simulink library "MainCANRX"  (R2015b)
settings: Solver=ode1  StartTime=0.0  StopTime=Inf  FixedStep=0.001  RelTol=1e-3
PostLoadFcn:
  | , if any(exist('dsrtsu_mdlpostloadfcn', 'file') == [2, 3, 6]), try dsrtsu_mdlpostloadfcn('Execute', bdroot); catch fprintf('Error in PostLoadFcn (dsrtsu_mdlpostloadfcn) for model "%s":\n %s\n', bdroot, lasterr); end, end,
libraries: rtican x4
settings Model: DSRTSU_INTERNAL_RTI_VER=460  DSRTSU_INTERNAL_RTI_TYPE=rti1401  Creator=luis  LastModifiedBy=luis
settings OptimizationCC: BlockReduction=off  OptimizeBlockIOStorage=off  BufferReuse=off  GlobalBufferReuse=off  ExpressionFolding=off  LocalBlockOutputs=off
settings HardwareCC: ProdEndianess=BigEndian  ProdWordSize=32  ProdHWDeviceType=Generic->Custom  TargetIntDivRoundTo=Zero  TargetEndianess=BigEndian  TargetHWDeviceType=Generic->Custom
settings RTWCC: SystemTargetFile=rti1401.tlc  MakeCommand=make_rti  TemplateMakefile=rti1401.tmf  Description=dSPACE DS1401 Hardware Platform
settings STFCustomTargetCC: ParMdlRefBuildCompliant=on  ConcurrentExecutionCompliant=off  GeneratePreprocessorConditionals=Use local settings  MatFileLogging=on  CPPClassGenCompliant=off  SystemTargetFile=rti1401.tlc
settings GRTTargetCC: CompOptLevelCompliant=off  ConcurrentExecutionCompliant=off  CombineOutputUpdateFcns=off  CPPClassGenCompliant=off  GRTInterface=on  UseToolchainInfoCompliant=off

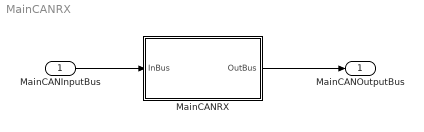
== system MainCANRX ==
  MainCANInputBus : Inport
  MainCANRX : Subsystem
  MainCANOutputBus : Outport
  wires:
  MainCANInputBus/1 -> MainCANRX/1(InBus)
  MainCANRX/1(OutBus) -> MainCANOutputBus/1

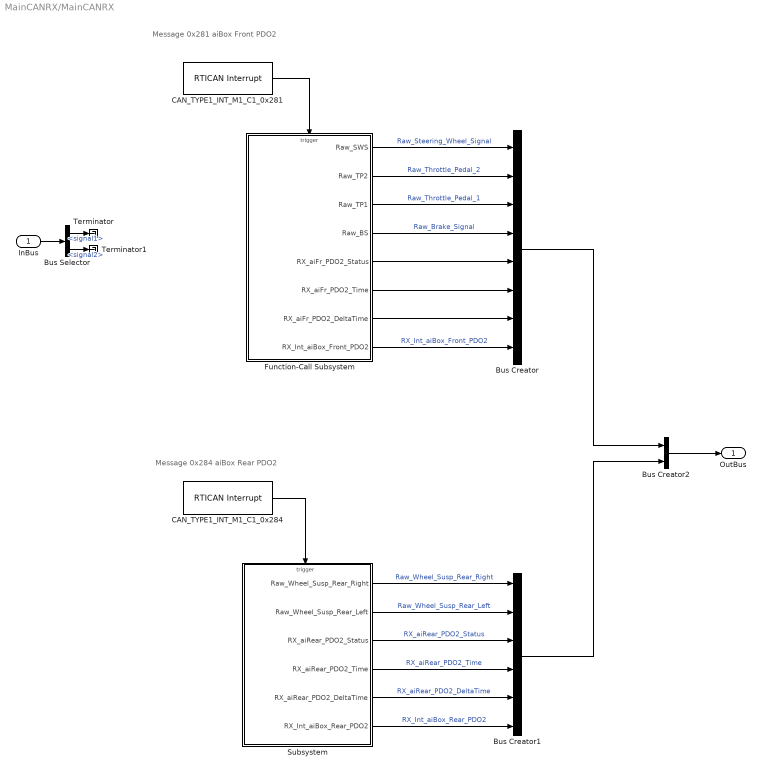
== system MainCANRX/MainCANRX ==
  note: Message 0x284 aiBox Rear PDO2
  note: Message 0x281 aiBox Front PDO2
  InBus : Inport
  Bus Creator : BusCreator  Inputs=8
  Bus Creator1 : BusCreator  Inputs=6
  Bus Creator2 : BusCreator  Inputs=2
  Bus Selector : BusSelector  OutputSignals=signal1,signal2
  CAN_TYPE1_INT_M1_C1_0x281 : rtican/RTICAN Interrupt  Reserved1=[]  Reserved2=[]  Reserved3=[]  Reserved4=[]  BoardTypeNo=[]  BoardNo=[]  ChannelNo=[]  Parameters=[]  InterruptName=[]  BoardIntNo=[]  Sfcn_Int_Struct=[]  BoardType=[]  SintNo=[]  Int_Struct=[]  DialogFcn=[]  UnitName=[]  Revision=[]  UnitValues=[]  DSProperties=struct('RTI',struct('Version',uint32(4),'BlockType',struct('isSLSource',uint8(1),'isSLSink',uint8(0),'isHWSource',uint8(1),'isHWSink',uint8(0),'isSetup',uint8(0),'isInline',uint8(1),'isNonInline',uint8(0),'isInterrupt',uint8(1),'isChannelwise',uint8(0)),'IOBoardType','RTICAN','UnitType','HWINT','Identifier','CANINT','DialogType','ML','BlockSet','RTICAN','RelationId',struct('TH',struct('BlockId','HWINT')),'SlaveProcessor','CAN'))  RTIBlockInterface=struct('OutputPortsWidth',int32(1),'FunctionCall',uint32(0),'OutputPortsActive',1,'DialogFcn','rtican_interrupt_gui','BlockDisplay',{{['CAN RX Interrupt'],'center'}},'IconTransparency','off','ParameterTunableNames',{{}},'InitLevel',3,'BlockName',struct('Token',{{'CAN_TYPE','_INT_M','_C'}},'BlockParam',{{'BoardTypeNo','BoardNo','ChannelNo'}}),'Options',{{'SS_OPTION_FORCE_NONINLINED_FCNCALL','SS_OPTION_ASYNCHRONOUS_INTERRUPT'}})  RTIBlockParameters=struct('BoardTypeNo',{{1,'OFF',[]}},'BoardNo',{{1,'ON',[1 16]}},'ChannelNo',{{1,'ON',[1 2]}},'Parameters',{{struct('general',struct('Type','RX','NumFormat','hex','MsgIdFormat','STD','MsgId',641,'isFromLib',0)),'OFF',[]}},'GroupId',{{struct('Group','RTICAN','No',1,'Behavior','NAMECHANGE','BlockType','SINK','NameChangeFlag',0),'OFF',[]}},'SFcnRTICANInterrupt',{{0,'OFF',[]}},'ThSrcSgnName',{{['CAN_TYPE1_M1_C1 RX Interrupt'],'OFF',[]}},'ThBlk',{{['struct(''blkh'',[''mainECU/MainCAN RX/CAN_TYPE1_INT_M1_C1_0x281''],''srcId'',''CAN1'',''srcSgnId'',''CAN1'',''intervalTmrBlockId'',[],''srcSgnName'',[''CAN_TYPE1_M1_C1 RX Interrupt''],''srcCpuId'','''',''isSrcCpu'',1,''isTargetCpu'',1,''srcOnMasterCpu'',1,''boardType'',''CAN'',''boardTypeNo'',''1'',''boardNo'',0,''intNo'',0,''subIntNo'',-1,''period'',0,''entryPoint'',''rti_CAN1'',''blockName'',''CAN_TYPE1_INT_M1_C1_0x281'',''taskNameDisplayExt'','''',''taskType'',''HWINT'',''groupId'',''CANINT1B1'',''hookFcn'',''NULL'',''isTimerTaskSrc'',0,''service'','''',''mpBlkId'','''',''taskPriorityPreConfig'',''none'',''taskPriority'',-1,''taskSortWeighting'',[],''taskSchedulingPolicy'',''FCFS'',''taskOvrPreConfig'',''none'',''taskOvrStrategy'',1,''taskOvrQueueSize'',1,''taskVisibility'',''on'',''taskGroupId'','''',''taskGroupDisplayOrder'',[],''serviceDynamicGen'',0,''disableCodeGen'',0,''boardBase'',''0'',''noBoardBase'','''')'],'OFF',[]}},'PHSBoardBaseId',{{'DS4302','OFF',[]}},'TLCFileName',{{'rtican_interrupt','OFF',[]}})  RTISFcnParameters=struct('SFcnRTICANInterrupt','struct','ThBlk','struct','PHSBoardBaseId','char','TLCFileName','char')  RTIBlockParaDefault=struct('BoardTypeNo',4302,'BoardNo',1,'ChannelNo',1,'Parameters',struct('general',struct('Type','RX','NumFormat','dec','MsgIdFormat','STD','MsgId',100,'isFromLib',1)),'GroupId',struct('Group',{{'RTICAN'}},'No',1,'Behavior',{{'NAMECHANGE'}},'BlockType',{{'SINK'}},'NameChangeFlag',0),'SFcnRTICANInterrupt',0,'ThSrcSgnName',['DS4302CAN_B1_C1 RX Interrupt'],'ThBlk',['struct(''srcSgnId'', '''')'],'PHSBoardBaseId','DS4302','TLCFileName','rtican_interrupt')
      settings: AttributesFormatString=Group Id: RTICAN1\n
  CAN_TYPE1_INT_M1_C1_0x284 : rtican/RTICAN Interrupt  Reserved1=[]  Reserved2=[]  Reserved3=[]  Reserved4=[]  BoardTypeNo=[]  BoardNo=[]  ChannelNo=[]  Parameters=[]  InterruptName=[]  BoardIntNo=[]  Sfcn_Int_Struct=[]  BoardType=[]  SintNo=[]  Int_Struct=[]  DialogFcn=[]  UnitName=[]  Revision=[]  UnitValues=[]  DSProperties=struct('RTI',struct('Version',uint32(4),'BlockType',struct('isSLSource',uint8(1),'isSLSink',uint8(0),'isHWSource',uint8(1),'isHWSink',uint8(0),'isSetup',uint8(0),'isInline',uint8(1),'isNonInline',uint8(0),'isInterrupt',uint8(1),'isChannelwise',uint8(0)),'IOBoardType','RTICAN','UnitType','HWINT','Identifier','CANINT','DialogType','ML','BlockSet','RTICAN','RelationId',struct('TH',struct('BlockId','HWINT')),'SlaveProcessor','CAN'))  RTIBlockInterface=struct('OutputPortsWidth',int32(1),'FunctionCall',uint32(0),'OutputPortsActive',1,'DialogFcn','rtican_interrupt_gui','BlockDisplay',{{['CAN RX Interrupt'],'center'}},'IconTransparency','off','ParameterTunableNames',{{}},'InitLevel',3,'BlockName',struct('Token',{{'CAN_TYPE','_INT_M','_C'}},'BlockParam',{{'BoardTypeNo','BoardNo','ChannelNo'}}),'Options',{{'SS_OPTION_FORCE_NONINLINED_FCNCALL','SS_OPTION_ASYNCHRONOUS_INTERRUPT'}})  RTIBlockParameters=struct('BoardTypeNo',{{1,'OFF',[]}},'BoardNo',{{1,'ON',[1 16]}},'ChannelNo',{{1,'ON',[1 2]}},'Parameters',{{struct('general',struct('Type','RX','NumFormat','hex','MsgIdFormat','STD','MsgId',644,'isFromLib',0)),'OFF',[]}},'GroupId',{{struct('Group','RTICAN','No',1,'Behavior','NAMECHANGE','BlockType','SINK','NameChangeFlag',0),'OFF',[]}},'SFcnRTICANInterrupt',{{0,'OFF',[]}},'ThSrcSgnName',{{['CAN_TYPE1_M1_C1 RX Interrupt'],'OFF',[]}},'ThBlk',{{['struct(''blkh'',[''mainECU/MainCAN RX/CAN_TYPE1_INT_M1_C1_0x284''],''srcId'',''CAN2'',''srcSgnId'',''CAN2'',''intervalTmrBlockId'',[],''srcSgnName'',[''CAN_TYPE1_M1_C1 RX Interrupt''],''srcCpuId'','''',''isSrcCpu'',1,''isTargetCpu'',1,''srcOnMasterCpu'',1,''boardType'',''CAN'',''boardTypeNo'',''1'',''boardNo'',0,''intNo'',1,''subIntNo'',-1,''period'',0,''entryPoint'',''rti_CAN2'',''blockName'',''CAN_TYPE1_INT_M1_C1_0x284'',''taskNameDisplayExt'','''',''taskType'',''HWINT'',''groupId'',''CANINT1B1'',''hookFcn'',''NULL'',''isTimerTaskSrc'',0,''service'','''',''mpBlkId'','''',''taskPriorityPreConfig'',''none'',''taskPriority'',-1,''taskSortWeighting'',[],''taskSchedulingPolicy'',''FCFS'',''taskOvrPreConfig'',''none'',''taskOvrStrategy'',1,''taskOvrQueueSize'',1,''taskVisibility'',''on'',''taskGroupId'','''',''taskGroupDisplayOrder'',[],''serviceDynamicGen'',0,''disableCodeGen'',0,''boardBase'',''0'',''noBoardBase'','''')'],'OFF',[]}},'PHSBoardBaseId',{{'DS4302','OFF',[]}},'TLCFileName',{{'rtican_interrupt','OFF',[]}})  RTISFcnParameters=struct('SFcnRTICANInterrupt','struct','ThBlk','struct','PHSBoardBaseId','char','TLCFileName','char')  RTIBlockParaDefault=struct('BoardTypeNo',4302,'BoardNo',1,'ChannelNo',1,'Parameters',struct('general',struct('Type','RX','NumFormat','dec','MsgIdFormat','STD','MsgId',100,'isFromLib',1)),'GroupId',struct('Group',{{'RTICAN'}},'No',1,'Behavior',{{'NAMECHANGE'}},'BlockType',{{'SINK'}},'NameChangeFlag',0),'SFcnRTICANInterrupt',0,'ThSrcSgnName',['DS4302CAN_B1_C1 RX Interrupt'],'ThBlk',['struct(''srcSgnId'', '''')'],'PHSBoardBaseId','DS4302','TLCFileName','rtican_interrupt')
      settings: AttributesFormatString=Group Id: RTICAN1\n
  Function-Call Subsystem : Subsystem  TreatAsAtomicUnit=on
  Subsystem : Subsystem
  Terminator : Terminator
  Terminator1 : Terminator
  OutBus : Outport
  wires:
  CAN_TYPE1_INT_M1_C1_0x281/1 -> Function-Call Subsystem/Trigger
  CAN_TYPE1_INT_M1_C1_0x284/1 -> Subsystem/Trigger
  Function-Call Subsystem/1(Raw_SWS) -> Bus Creator/1  "Raw_Steering_Wheel_Signal"
  Subsystem/6(RX_Int_aiBox_Rear_PDO2) -> Bus Creator1/6  "RX_Int_aiBox_Rear_PDO2"
  Subsystem/1(Raw_Wheel_Susp_Rear_Right) -> Bus Creator1/1  "Raw_Wheel_Susp_Rear_Right"
  Function-Call Subsystem/8(RX_Int_aiBox_Front_PDO2) -> Bus Creator/8  "RX_Int_aiBox_Front_PDO2"
  Subsystem/3(RX_aiRear_PDO2_Status) -> Bus Creator1/3  "RX_aiRear_PDO2_Status"
  Function-Call Subsystem/3(Raw_TP1) -> Bus Creator/3  "Raw_Throttle_Pedal_1"
  Function-Call Subsystem/7(RX_aiFr_PDO2_DeltaTime) -> Bus Creator/7
  Function-Call Subsystem/6(RX_aiFr_PDO2_Time) -> Bus Creator/6
  Function-Call Subsystem/4("Raw_BS ") -> Bus Creator/4  "Raw_Brake_Signal"
  Subsystem/4(RX_aiRear_PDO2_Time) -> Bus Creator1/4  "RX_aiRear_PDO2_Time"
  Subsystem/2(Raw_Wheel_Susp_Rear_Left) -> Bus Creator1/2  "Raw_Wheel_Susp_Rear_Left"
  Function-Call Subsystem/5(RX_aiFr_PDO2_Status) -> Bus Creator/5
  Function-Call Subsystem/2(Raw_TP2) -> Bus Creator/2  "Raw_Throttle_Pedal_2"
  Subsystem/5(RX_aiRear_PDO2_DeltaTime) -> Bus Creator1/5  "RX_aiRear_PDO2_DeltaTime"
  Bus Selector/1 -> Terminator/1  "<signal1>"
  InBus/1 -> Bus Selector/1
  Bus Creator/1 -> Bus Creator2/1
  Bus Creator1/1 -> Bus Creator2/2
  Bus Creator2/1 -> OutBus/1
  Bus Selector/2 -> Terminator1/1  "<signal2>"

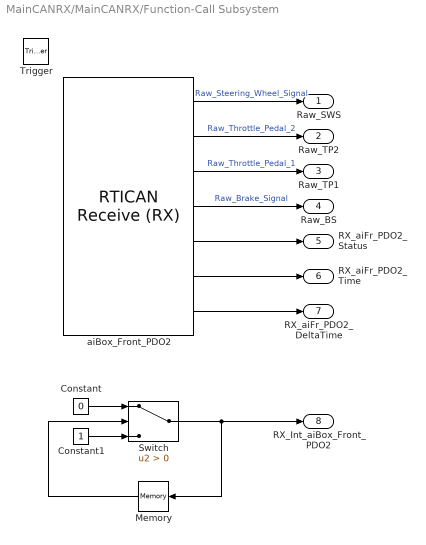
== system MainCANRX/MainCANRX/Function-Call Subsystem ==
  Trigger : TriggerPort  TriggerType=function-call  OutputDataType=double
  Constant : Constant  Value=0
  Constant1 : Constant
  Memory : Memory  InheritSampleTime=on
  Switch : Switch  Criteria=u2 > Threshold
  aiBox_Front_PDO2 : rtican/RTICAN Receive (RX)   Reserved1=[]  Reserved2=[]  Reserved3=[]  Reserved4=[]  SfcnMessage=[]  Msg_Struct=[]  BoardTypeNo=[]  BoardNo=[]  ChannelNo=[]  Parameters=[]  DialogFcn=[]  UnitName=[]  Revision=[]  UnitValues=[]  DSProperties=struct('RTI',struct('Version',uint32(5),'BlockType',struct('isSLSource',uint8(1),'isSLSink',uint8(1),'isHWSource',uint8(0),'isHWSink',uint8(0),'isSetup',uint8(0),'isInline',uint8(1),'isNonInline',uint8(0),'isInterrupt',uint8(0),'isChannelwise',uint8(0)),'IOBoardType','RTICAN','UnitType','MESSAGE','Identifier','RX','DialogType','MSVC','BlockSet','RTICAN','SlaveProcessor','CAN'))  RTIBlockInterface=struct('OutputPortsWidth',int32([1 1 1 1 1 1 1]),'OutputPortsActive',[1 1 1 1 1 1 1],'OutputPortsName',{{'Raw_Steering_Wheel_Signal','Raw_Throttle_Pedal_2','Raw_Throttle_Pedal_1','Raw_Brake_Signal',['RX status'],['RX time'],['RX delta time']}},'OutputPortsDataType',{{'SS_DOUBLE','SS_DOUBLE','SS_DOUBLE','SS_DOUBLE','SS_DOUBLE','SS_DOUBLE','SS_DOUBLE'}},'OutputPortsLabel',{{'Raw_Steering_Wheel_Signal','Raw_Throttle_Pedal_2','Raw_Throttle_Pedal_1','Raw_Brake_Signal','','',''}},'OutputPortsLabelMode','ON','InputPortsWidth',int32(0),'InputPortsActive',0,'DialogFcn','rtican_message_interface_gui','BlockDisplay',{{'','center'}},'IconTransparency','on','ParameterTunableNames',{{}},'InitLevel',3,'BlockName',struct('Token',{{'aiBox_Front_PDO2'}}),'SampleTime',{{-1}},'TriggerPort',{{'none'}},'EnablePort',{{'none'}})  RTIBlockParameters=struct('BoardTypeNo',{{1,'OFF',[]}},'BoardNo',{{1,'ON',[1 16]}},'ChannelNo',{{1,'ON',[1 2]}},'Parameters',{{struct('DataFileSupport',struct('DataFileSelectedMaster',1,'DataFileSelectedLocal',1,'DataFileName',['c:\users\luis\documents\tuc racing\mainecu\database\main_0_2.dbc|'],'DataFileDate',{{{['07-ene.-2017 20:06:27']}}},'SelectedFile','database\main_0_2.dbc'),'Options',struct('StatusSelected',1,'TimeSelected',1,'DeltaTimeSelected',1,'BytePortSelected',0,'MessageLengthSelected',0,'TriggerPort',struct('Selected',0,'TriggerType',0),'UserCoding',struct('Selected',0,'InterfaceFile','UserDecodingFile','FcnName','UserDecodeFcn','InportSelected',0,'InportWidth',1,'OutportSelected',0,'OutportWidth',1),'EnablePortSelected',0,'SignalOnPortnameSelected',1,'UseRXService',0),'Message',struct('MsgOnBlocknameSelected',1,'MsgName','aiBox_Front_PDO2','MsgIdFormat',0,'MsgId',641,'MsgLength',8,'NumSignals',4,'SampleTime',-1,'Signal',struct('SgnName',{'Raw_Steering_Wheel_Signal','Raw_Throttle_Pedal_2','Raw_Throttle_Pedal_1','Raw_Brake_Signal'},'SgnStartBit',{0,16,32,48},'SgnLength',{16,16,16,16},'SgnType',{0,0,0,0},'ModeValue',{-1,-1,-1,-1},'DataType',{0,0,0,0},'ByteLayout',{2,2,2,2},'Factor',{1,1,1,1},'Offset',{0,0,0,0},'SgnComment',{{''},{''},{''},{''}},'SgnUnit',{'','','',''},'Min',{0,0,0,0},'Max',{0,0,0,0},'SLDataType',{'SS_DOUBLE','SS_DOUBLE','SS_DOUBLE','SS_DOUBLE'}),'MsgIdNumFormat',1,'MsgComment',{{''}}),'Version',1.2,'general',struct('isFromLib',0)),'OFF',[]}},'GroupId',{{struct('Group',{{'RTICAN'}},'No',1,'Behavior',{{'NAMECHANGE'}},'BlockType',{{'SINK'}},'NameChangeFlag',0),'OFF',[]}},'SFcnRTICANMessage',{{struct('MsgType','RX','SFcnPortType','Scalar','MsgName','aiBox_Front_PDO2','MsgIdFormat','STD','MsgId',641,'MsgLength',8,'NumSignals',4,'SampleTime',-1,'Signal',struct('SgnName',{'Raw_Steering_Wheel_Signal','Raw_Throttle_Pedal_2','Raw_Throttle_Pedal_1','Raw_Brake_Signal'},'SgnStartBit',{0,16,32,48},'SgnLength',{16,16,16,16},'SgnType',{'standard','standard','standard','standard'},'ModeValue',{-1,-1,-1,-1},'DataType',{['unsigned int'],['unsigned int'],['unsigned int'],['unsigned int']},'ByteLayout',{['motorola back.'],['motorola back.'],['motorola back.'],['motorola back.']},'Factor',{1,1,1,1},'Offset',{0,0,0,0},'SLDataType',{'SS_DOUBLE','SS_DOUBLE','SS_DOUBLE','SS_DOUBLE'}),'StatusSelected','yes','TimeSelected','yes','DeltaTimeSelected','yes','BytePortSelected','no','MessageLengthSelected','no','TriggerPort',struct('Selected','no','TriggerType',0),'UserCoding',struct('Selected','no','InterfaceFile','UserDecodingFile','FcnName','UserDecodeFcn','InportSelected','no','InportWidth',1,'OutportSelected','no','OutportWidth',1),'EnablePortSelected','no','UseRXService','no','BoardType','DS1','BoardNo',1,'ControllerNo',1),'OFF',[]}},'TLCFileName',{{'rtican_rx_message','OFF',[]}})  RTISFcnParameters=struct('SFcnRTICANMessage','struct','TLCFileName','char')  RTIBlockParaDefault=struct('BoardTypeNo',4302,'BoardNo',1,'ChannelNo',1,'Parameters',struct('DataFileSupport',struct('DataFileSelectedMaster',0,'DataFileSelectedLocal',0,'DataFileName','','DataFileDate','','SelectedFile',['<no file selected>']),'Options',struct('StatusSelected',1,'TimeSelected',1,'DeltaTimeSelected',1,'BytePortSelected',0,'MessageLengthSelected',0,'TriggerPort',struct('Selected',0,'TriggerType','rising'),'UserCoding',struct('Selected',0,'InterfaceFile','UserDecodingFile','FcnName','UserDecodeFcn','InportSelected',0,'InportWidth',1,'OutportSelected',0,'OutportWidth',1),'EnablePortSelected',0,'SignalOnPortnameSelected',1,'UseRXService',0),'Message',struct('MsgOnBlocknameSelected',0,'MsgName',['RX Message'],'MsgIdFormat',0,'MsgId',100,'MsgLength',8,'NumSignals',1,'SampleTime',-1,'Signal',struct('SgnName',['RX signal'],'SgnStartBit',0,'SgnLength',8,'SgnType',0,'ModeValue',-1,'DataType',0,'SLDataType','SS_DOUBLE','ByteLayout',0,'Factor',1,'Offset',0,'Min',0,'Max',255,'SgnComment',{{}},'SgnUnit',''),'MsgIdNumFormat',0,'MsgComment',{{''}}),'Version',1.2,'general',struct('isFromLib',1)),'GroupId',struct('Group',{{'RTICAN'}},'No',1,'Behavior',{{'NAMECHANGE'}},'BlockType',{{'SINK'}},'NameChangeFlag',0),'SFcnRTICANMessage',struct('MsgType','RX','MsgName',['RX Message'],'MsgIdFormat','STD','MsgId',100,'MsgLength',8,'NumSignals',1,'SampleTime',-1,'Signal',struct('SgnName',['RX signal'],'SgnStartBit',0,'SgnLength',8,'SgnType','standard','ModeValue',-1,'DataType',['unsigned int'],'ByteLayout',['little endian'],'SLDataType','SS_DOUBLE','Factor',1,'Offset',0),'StatusSelected','yes','TimeSelected','yes','DeltaTimeSelected','yes','BytePortSelected','no','MessageLengthSelected','no','EnablePortSelected','no','UserCoding',struct('Selected','no','InterfaceFile','UserDecodingFile','FcnName','UserDecodeFcn','InportSelected','no','InportWidth',1,'OutportSelected','no','OutportWidth',1),'TriggerPort',struct('Selected','no','TriggerType','rising'),'UseRXService','no','BoardType','DS4302','BoardNo',1,'ControllerNo',1,'SFcnPortType','Scalar'),'TLCFileName','rtican_rx_message')
      settings: AttributesFormatString=Group Id: RTICAN1\n
  Raw_SWS : Outport
  Raw_TP2 : Outport  Port=2
  Raw_TP1 : Outport  Port=3
  "Raw_BS " : Outport  Port=4
  RX_aiFr_PDO2_Status : Outport  Port=5
  RX_aiFr_PDO2_Time : Outport  Port=6
  RX_aiFr_PDO2_DeltaTime : Outport  Port=7
  RX_Int_aiBox_Front_PDO2 : Outport  Port=8
  wires:
  aiBox_Front_PDO2/1 -> Raw_SWS/1  "Raw_Steering_Wheel_Signal"
  aiBox_Front_PDO2/2 -> Raw_TP2/1  "Raw_Throttle_Pedal_2"
  aiBox_Front_PDO2/3 -> Raw_TP1/1  "Raw_Throttle_Pedal_1"
  aiBox_Front_PDO2/4 -> "Raw_BS "/1  "Raw_Brake_Signal"
  aiBox_Front_PDO2/5 -> RX_aiFr_PDO2_Status/1
  aiBox_Front_PDO2/6 -> RX_aiFr_PDO2_Time/1
  aiBox_Front_PDO2/7 -> RX_aiFr_PDO2_DeltaTime/1
  Switch/1 -> Memory/1, RX_Int_aiBox_Front_PDO2/1
  Memory/1 -> Switch/2
  Constant1/1 -> Switch/3
  Constant/1 -> Switch/1

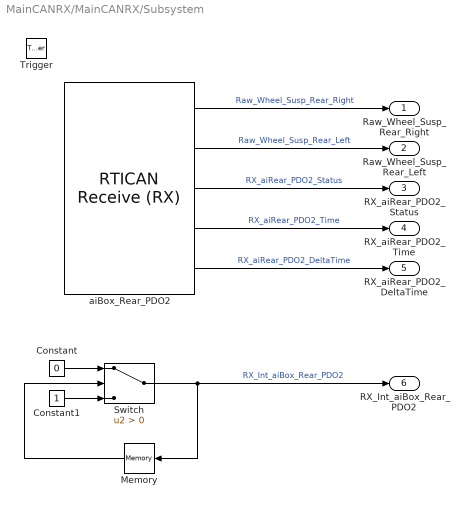
== system MainCANRX/MainCANRX/Subsystem ==
  Trigger : TriggerPort  TriggerType=function-call  PortDimensions=1
  Constant : Constant  Value=0
  Constant1 : Constant
  Memory : Memory  InheritSampleTime=on
  Switch : Switch  Criteria=u2 > Threshold
  aiBox_Rear_PDO2 : rtican/RTICAN Receive (RX)   Reserved1=[]  Reserved2=[]  Reserved3=[]  Reserved4=[]  SfcnMessage=[]  Msg_Struct=[]  BoardTypeNo=[]  BoardNo=[]  ChannelNo=[]  Parameters=[]  DialogFcn=[]  UnitName=[]  Revision=[]  UnitValues=[]  DSProperties=struct('RTI',struct('Version',uint32(5),'BlockType',struct('isSLSource',uint8(1),'isSLSink',uint8(1),'isHWSource',uint8(0),'isHWSink',uint8(0),'isSetup',uint8(0),'isInline',uint8(1),'isNonInline',uint8(0),'isInterrupt',uint8(0),'isChannelwise',uint8(0)),'IOBoardType','RTICAN','UnitType','MESSAGE','Identifier','RX','DialogType','MSVC','BlockSet','RTICAN','SlaveProcessor','CAN'))  RTIBlockInterface=struct('OutputPortsWidth',int32([1 1 1 1 1]),'OutputPortsActive',[1 1 1 1 1],'OutputPortsName',{{'Raw_Wheel_Susp_Rear_Right','Raw_Wheel_Susp_Rear_Left',['RX status'],['RX time'],['RX delta time']}},'OutputPortsDataType',{{'SS_DOUBLE','SS_DOUBLE','SS_DOUBLE','SS_DOUBLE','SS_DOUBLE'}},'OutputPortsLabel',{{'Raw_Wheel_Susp_Rear_Right','Raw_Wheel_Susp_Rear_Left','','',''}},'OutputPortsLabelMode','ON','InputPortsWidth',int32(0),'InputPortsActive',0,'DialogFcn','rtican_message_interface_gui','BlockDisplay',{{'','center'}},'IconTransparency','on','ParameterTunableNames',{{}},'InitLevel',3,'BlockName',struct('Token',{{'aiBox_Rear_PDO2'}}),'SampleTime',{{-1}},'TriggerPort',{{'none'}},'EnablePort',{{'none'}})  RTIBlockParameters=struct('BoardTypeNo',{{1,'OFF',[]}},'BoardNo',{{1,'ON',[1 16]}},'ChannelNo',{{1,'ON',[1 2]}},'Parameters',{{struct('DataFileSupport',struct('DataFileSelectedMaster',1,'DataFileSelectedLocal',1,'DataFileName',['c:\users\luis\documents\tuc racing\mainecu\database\main_0_2.dbc|'],'DataFileDate',{{{['07-ene.-2017 20:06:27']}}},'SelectedFile','database\main_0_2.dbc'),'Options',struct('StatusSelected',1,'TimeSelected',1,'DeltaTimeSelected',1,'BytePortSelected',0,'MessageLengthSelected',0,'TriggerPort',struct('Selected',0,'TriggerType',0),'UserCoding',struct('Selected',0,'InterfaceFile','UserDecodingFile','FcnName','UserDecodeFcn','InportSelected',0,'InportWidth',1,'OutportSelected',0,'OutportWidth',1),'EnablePortSelected',0,'SignalOnPortnameSelected',1,'UseRXService',0),'Message',struct('MsgOnBlocknameSelected',1,'MsgName','aiBox_Rear_PDO2','MsgIdFormat',0,'MsgId',644,'MsgLength',8,'NumSignals',2,'SampleTime',-1,'Signal',struct('SgnName',{'Raw_Wheel_Susp_Rear_Right','Raw_Wheel_Susp_Rear_Left'},'SgnStartBit',{32,48},'SgnLength',{16,16},'SgnType',{0,0},'ModeValue',{-1,-1},'DataType',{0,0},'ByteLayout',{2,2},'Factor',{1,1},'Offset',{0,0},'SgnComment',{{''},{''}},'SgnUnit',{'',''},'Min',{0,0},'Max',{0,0},'SLDataType',{'SS_DOUBLE','SS_DOUBLE'}),'MsgIdNumFormat',0,'MsgComment',{{''}}),'Version',1.2,'general',struct('isFromLib',0)),'OFF',[]}},'GroupId',{{struct('Group',{{'RTICAN'}},'No',1,'Behavior',{{'NAMECHANGE'}},'BlockType',{{'SINK'}},'NameChangeFlag',0),'OFF',[]}},'SFcnRTICANMessage',{{struct('MsgType','RX','SFcnPortType','Scalar','MsgName','aiBox_Rear_PDO2','MsgIdFormat','STD','MsgId',644,'MsgLength',8,'NumSignals',2,'SampleTime',-1,'Signal',struct('SgnName',{'Raw_Wheel_Susp_Rear_Right','Raw_Wheel_Susp_Rear_Left'},'SgnStartBit',{32,48},'SgnLength',{16,16},'SgnType',{'standard','standard'},'ModeValue',{-1,-1},'DataType',{['unsigned int'],['unsigned int']},'ByteLayout',{['motorola back.'],['motorola back.']},'Factor',{1,1},'Offset',{0,0},'SLDataType',{'SS_DOUBLE','SS_DOUBLE'}),'StatusSelected','yes','TimeSelected','yes','DeltaTimeSelected','yes','BytePortSelected','no','MessageLengthSelected','no','TriggerPort',struct('Selected','no','TriggerType',0),'UserCoding',struct('Selected','no','InterfaceFile','UserDecodingFile','FcnName','UserDecodeFcn','InportSelected','no','InportWidth',1,'OutportSelected','no','OutportWidth',1),'EnablePortSelected','no','UseRXService','no','BoardType','DS1','BoardNo',1,'ControllerNo',1),'OFF',[]}},'TLCFileName',{{'rtican_rx_message','OFF',[]}})  RTISFcnParameters=struct('SFcnRTICANMessage','struct','TLCFileName','char')  RTIBlockParaDefault=struct('BoardTypeNo',4302,'BoardNo',1,'ChannelNo',1,'Parameters',struct('DataFileSupport',struct('DataFileSelectedMaster',0,'DataFileSelectedLocal',0,'DataFileName','','DataFileDate','','SelectedFile',['<no file selected>']),'Options',struct('StatusSelected',1,'TimeSelected',1,'DeltaTimeSelected',1,'BytePortSelected',0,'MessageLengthSelected',0,'TriggerPort',struct('Selected',0,'TriggerType','rising'),'UserCoding',struct('Selected',0,'InterfaceFile','UserDecodingFile','FcnName','UserDecodeFcn','InportSelected',0,'InportWidth',1,'OutportSelected',0,'OutportWidth',1),'EnablePortSelected',0,'SignalOnPortnameSelected',1,'UseRXService',0),'Message',struct('MsgOnBlocknameSelected',0,'MsgName',['RX Message'],'MsgIdFormat',0,'MsgId',100,'MsgLength',8,'NumSignals',1,'SampleTime',-1,'Signal',struct('SgnName',['RX signal'],'SgnStartBit',0,'SgnLength',8,'SgnType',0,'ModeValue',-1,'DataType',0,'SLDataType','SS_DOUBLE','ByteLayout',0,'Factor',1,'Offset',0,'Min',0,'Max',255,'SgnComment',{{}},'SgnUnit',''),'MsgIdNumFormat',0,'MsgComment',{{''}}),'Version',1.2,'general',struct('isFromLib',1)),'GroupId',struct('Group',{{'RTICAN'}},'No',1,'Behavior',{{'NAMECHANGE'}},'BlockType',{{'SINK'}},'NameChangeFlag',0),'SFcnRTICANMessage',struct('MsgType','RX','MsgName',['RX Message'],'MsgIdFormat','STD','MsgId',100,'MsgLength',8,'NumSignals',1,'SampleTime',-1,'Signal',struct('SgnName',['RX signal'],'SgnStartBit',0,'SgnLength',8,'SgnType','standard','ModeValue',-1,'DataType',['unsigned int'],'ByteLayout',['little endian'],'SLDataType','SS_DOUBLE','Factor',1,'Offset',0),'StatusSelected','yes','TimeSelected','yes','DeltaTimeSelected','yes','BytePortSelected','no','MessageLengthSelected','no','EnablePortSelected','no','UserCoding',struct('Selected','no','InterfaceFile','UserDecodingFile','FcnName','UserDecodeFcn','InportSelected','no','InportWidth',1,'OutportSelected','no','OutportWidth',1),'TriggerPort',struct('Selected','no','TriggerType','rising'),'UseRXService','no','BoardType','DS4302','BoardNo',1,'ControllerNo',1,'SFcnPortType','Scalar'),'TLCFileName','rtican_rx_message')
      settings: AttributesFormatString=Group Id: RTICAN1\n
  Raw_Wheel_Susp_Rear_Right : Outport
  Raw_Wheel_Susp_Rear_Left : Outport  Port=2
  RX_aiRear_PDO2_Status : Outport  Port=3
  RX_aiRear_PDO2_Time : Outport  Port=4
  RX_aiRear_PDO2_DeltaTime : Outport  Port=5
  RX_Int_aiBox_Rear_PDO2 : Outport  Port=6
  wires:
  aiBox_Rear_PDO2/1 -> Raw_Wheel_Susp_Rear_Right/1  "Raw_Wheel_Susp_Rear_Right"
  aiBox_Rear_PDO2/5 -> RX_aiRear_PDO2_DeltaTime/1  "RX_aiRear_PDO2_DeltaTime"
  aiBox_Rear_PDO2/3 -> RX_aiRear_PDO2_Status/1  "RX_aiRear_PDO2_Status"
  aiBox_Rear_PDO2/2 -> Raw_Wheel_Susp_Rear_Left/1  "Raw_Wheel_Susp_Rear_Left"
  aiBox_Rear_PDO2/4 -> RX_aiRear_PDO2_Time/1  "RX_aiRear_PDO2_Time"
  Switch/1 -> Memory/1, RX_Int_aiBox_Rear_PDO2/1  "RX_Int_aiBox_Rear_PDO2"
  Memory/1 -> Switch/2
  Constant1/1 -> Switch/3
  Constant/1 -> Switch/1
